simulink model "statemdemo"  (Simulink 8.0)
settings: Solver=ode45  StartTime=0.0  StopTime=inf  RelTol=1e-3
settings Model: Creator=caster  LastModifiedBy=caster

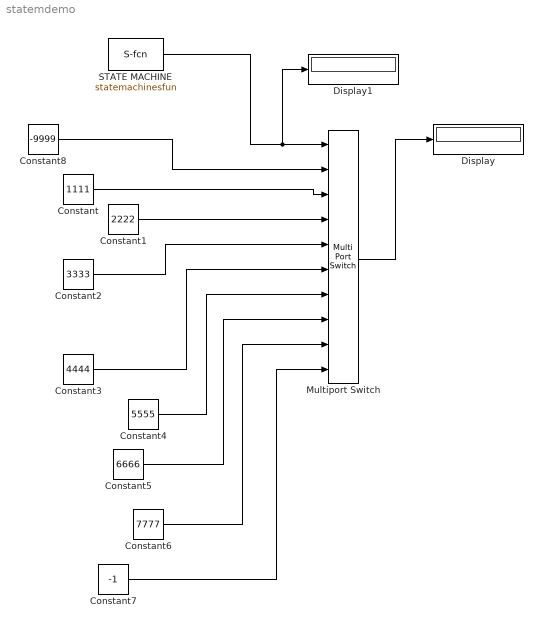
== system statemdemo ==
  Constant : Constant  Value=1111
  Constant1 : Constant  Value=2222
  Constant2 : Constant  Value=3333
  Constant3 : Constant  Value=4444
  Constant4 : Constant  Value=5555
  Constant5 : Constant  Value=6666
  Constant6 : Constant  Value=7777
  Constant7 : Constant  Value=-1
  Constant8 : Constant  Value=-9999
  Display : Display
  Display1 : Display
  Multiport Switch : MultiPortSwitch  DataPortOrder=Zero-based contiguous  Inputs=9
  STATE MACHINE : M-S-Function  FunctionName=statemachinesfun
  wires:
  STATE MACHINE/1 -> Display1/1, Multiport Switch/1
  Constant/1 -> Multiport Switch/3
  Constant1/1 -> Multiport Switch/4
  Constant2/1 -> Multiport Switch/5
  Constant3/1 -> Multiport Switch/6
  Constant4/1 -> Multiport Switch/7
  Constant5/1 -> Multiport Switch/8
  Constant6/1 -> Multiport Switch/9
  Constant7/1 -> Multiport Switch/10
  Multiport Switch/1 -> Display/1
  Constant8/1 -> Multiport Switch/2
